simulink model "Exp10"  (R2018a)
settings: Solver=ode23tb  StartTime=0.0  StopTime=0.4  RelTol=1e-4
libraries: powerlib x31
Description:
  | Copyright 2008-2018 The MathWorks, Inc.
settings Model: ExtModeTrigMode=oneshot  ExtModeArmWhenConnect=off  ExtModeAutoUpdateStatusClock=off  Creator=MathWorks  LastModifiedBy=Asus
settings DataIOCC: ExternalInput=[]  SaveFormat=Array  SignalLoggingSaveFormat=ModelDataLogs  SaveOutput=off  SignalLoggingName=sigsOut
settings OptimizationCC: BlockReduction=off  BooleanDataType=off  ExpressionDepthLimit=2147483647  InitFltsAndDblsToZero=on  EfficientMapNaN2IntZero=off  LifeSpan=inf
settings DebuggingCC: AlgebraicLoopMsg=none  UnderspecifiedInitializationDetection=Classic  MergeDetectMultiDrivingBlocksExec=none  CheckExecutionContextPreStartOutputMsg=on  CheckExecutionContextRuntimeOutputMsg=on  SignalResolutionControl=TryResolveAllWithWarning  MultiTaskDSMMsg=warning  MultiTaskCondExecSysMsg=none  SigSpecEnsureSampleTimeMsg=none  FcnCallInpInsideContextMsg=warning  StateNameClashWarn=warning  SFUnexpectedBacktrackingDiag=warning  SFNoUnconditionalDefaultTransitionDiag=warning  SFExecutionAtInitializationDiag=none
settings HardwareCC: ProdBitPerPointer=32  ProdBitPerSizeT=32  ProdBitPerPtrDiffT=32  ProdLargestAtomicFloat=None  ProdIntDivRoundTo=Undefined  ProdEndianess=Unspecified  ProdWordSize=32  ProdHWDeviceType=32-bit Generic  TargetUnknown=on
settings ModelReferenceCC: PropagateSignalLabelsOutOfModel=off
settings CodeAppCC: StateflowObjectComments=on
settings GRTTargetCC: TargetLangStandard=C89/C90 (ANSI)  GeneratePreprocessorConditionals=Disable all  CombineOutputUpdateFcns=off  GRTInterface=on
settings ConfigComp: CovMetricSettings=dw  CovHtmlReporting=on  CovSaveCumulativeToWorkspaceVar=on  CovSaveSingleToWorkspaceVar=on  CovExternalEMLEnable=off  CovSFcnEnable=off
settings SimscapeCC: SimscapeNormalizeSystem=off

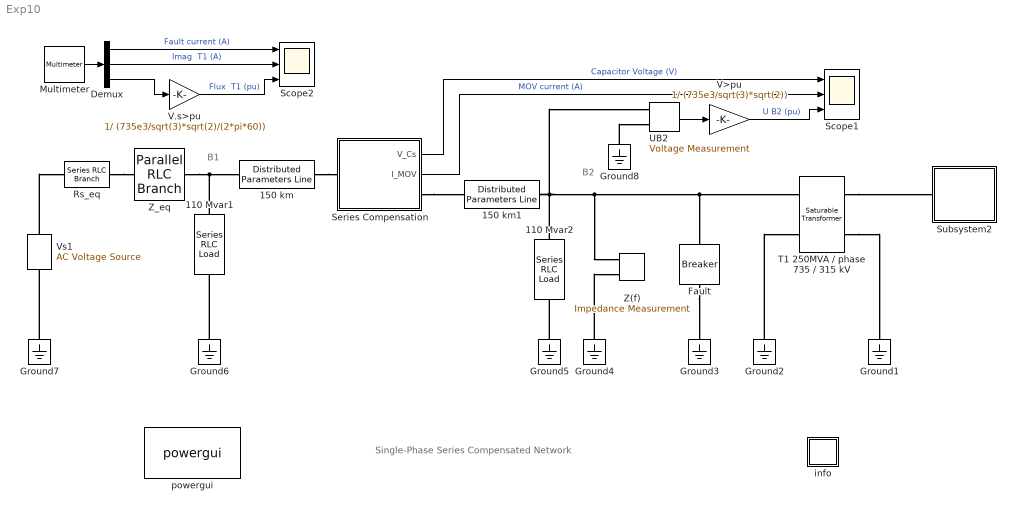
== system Exp10 ==
  note: Single-Phase Series Compensated Network
  note: B1
  note: B2
  110 Mvar1 : powerlib/Elements/Series RLC Load  LConnTagsString=a  RConnTagsString=__new0  NominalVoltage=735000/sqrt(3)  NominalFrequency=60  ActivePower=110e6/300  InductivePower=110e6  CapacitivePower=0  Setx0=off  InitialVoltage=0  SetiL0=off  InitialCurrent=0  Measurements=None  LoadType=constant Z
  110 Mvar2 : powerlib/Elements/Series RLC Load  LConnTagsString=a  RConnTagsString=__new0  NominalVoltage=735000/sqrt(3)  NominalFrequency=60  ActivePower=110e6/300  InductivePower=110e6  CapacitivePower=0  Setx0=off  InitialVoltage=0  SetiL0=off  InitialCurrent=0  Measurements=None  LoadType=constant Z
  150 km : powerlib/Elements/Distributed Parameters Line  Phases=1  Frequency=60  Resistance=0.011  Inductance=0.8674e-03  Capacitance=13.41e-09  Length=150  x1=[602382.210728082;376.991118430775;-0.201832804872111]  x2=[617832.687776944;376.991118430775;-0.223349800057888]  x3=[2166.90364173997;376.991118430775;-0.458497477125126]  x4=[2673.14981372514;376.991118430775;-0.188540324238639]  x5=0.000511582119507709  V1=[6.024e+05;377;-0.2018]  V2=[6.178e+05;377;-0.2233]  I1=[2167;377;-0.4585]  I2=[2673;377;-0.1885]  nHarmo=1  Measurements=None
      settings: AttributesFormatString=\n  SourceProductName=Simscape Power Systems
  150 km1 : powerlib/Elements/Distributed Parameters Line  Phases=1  Frequency=60  Resistance=0.011  Inductance=0.8674e-03  Capacitance=13.41e-09  Length=150  x1=[614251.726505356;376.991118430775;-0.207067226534412]  x2=[606916.918046152;376.991118430775;-0.227269187006359]  x3=[2149.77581818931;376.991118430775;-0.248424449769665]  x4=[2658.79697353536;376.991118430775;-0.366457341038554]  x5=0.000511582119507709  V1=[6.143e+05;377;-0.2071]  V2=[6.069e+05;377;-0.2273]  I1=[2150;377;-0.2484]  I2=[2659;377;-0.3665]  nHarmo=1  Measurements=None
      settings: AttributesFormatString=\n  SourceProductName=Simscape Power Systems
  Demux : Demux  Outputs=3
  Fault : powerlib/Elements/Breaker  InitialState=0  SwitchingTimes="[ 3/60  9/60 ]"  External=off  BreakerResistance=0.01  SnubberResistance=inf  SnubberCapacitance=0  Measurements=Branch current  MoreParameters=off  NoBreakLoop=off
      settings: AttributesFormatString=\n  SourceProductName=Simscape Power Systems
  Ground{1..8} (8 alike) : powerlib/Elements/Ground  LConnTagsString=a
  Multimeter : powerlib/Measurements/Multimeter  Tag=PoWeRsYsTeMmEaSuReMeNt  PhasorSimulation=off  OutputType=Magnitude  sel=[1 3 4]  L=4  Gain=[1 1 1]  yselected="{'Ib: Fault','Imag: T1  250MVA // phase  735 // 315 kV','Flux: T1  250MVA // phase  735 // 315 kV'};"  PSBOutputType=1  PSBequivalent=0  AxesSetting=[0,0.1,-100,100]  Display=0  SavedBlockNames={}
      settings: AttributesFormatString=\n
  Rs_eq : powerlib/Elements/Series RLC Branch  LConnTagsString=__new0  RConnTagsString=__new0  BranchType=R  Resistance=2  Inductance=[]  SetiL0=off  InitialCurrent=0  Capacitance=[]  Setx0=off  InitialVoltage=0  Measurements=None
  Scope1 : Scope  NumInputPorts=3
  Scope2 : Scope  NumInputPorts=3
  Series Compensation : Subsystem
      mask Display: plot(0,0,100,100,[10 40],[50 50], [40 40],[40 60],[60 60],[40 60], [60 90],[50 50])
  Subsystem2 : Subsystem
      mask Display: disp('315 kV\nEquivalent')
  T1 250MVA / phase 735 / 315 kV : powerlib/Elements/Saturable Transformer  ThreeWindings=off  Hysteresis=off  DataFile='hysteresis'  Measurements=Flux and magnetization current ( Imag )  UNITS=pu  NominalPower=[750e6/3,60]  Winding1=[735000/sqrt(3), 0.001 ,0.15]  Winding2=[315000/sqrt(3), 0.001,0]  Winding3=[315000/sqrt(3), 0.001,0]  Saturation=[0 0 ; 0.0012 1.2; 1.0 1.45 ]  CoreLoss=[1000]  MoreParameters=off  BreakLoop=off  DataType=off  InitialFlux=-1606.09832312951  TransfoNumber=1
      settings: AttributesFormatString=\n  SourceProductName=Simscape Power Systems  SourceProductBaseCode=PS
  UB2 : powerlib/Measurements/Voltage Measurement  Tag=PoWeRsYsTeMmEaSuReMeNt  PhasorSimulation=off  OutputType=Magnitude  PSBequivalent=0
  V.s>pu : Gain  Gain=1/ (735e3/sqrt(3)*sqrt(2)/(2*pi*60))  SaturateOnIntegerOverflow=on  OutDataTypeStr=Inherit: Same as input  ParamDataTypeStr=Inherit: Same as input
  V>pu : Gain  Gain=1/ (735e3/sqrt(3)*sqrt(2))  SaturateOnIntegerOverflow=on  OutDataTypeStr=Inherit: Same as input  ParamDataTypeStr=Inherit: Same as input
  Vs1 : powerlib/Electrical Sources/AC Voltage Source  Description=source block  Amplitude=735000/sqrt(3)*sqrt(2)  Phase=0  Frequency=60  SampleTime=0  Measurements=None  BusType=swing  Pref=10e3  Qref=0  Qmin=-inf  Qmax=+inf
      settings: AttributesFormatString=\n
  Z(f) : powerlib/Measurements/Impedance Measurement  LConnTagsString=+|-  Factor=1
      settings: AttributesFormatString=\n  SourceProductName=Simscape Power Systems  SourceProductBaseCode=PS
  Z_eq : powerlib/Elements/Parallel RLC Branch  LConnTagsString=a  RConnTagsString=__new0  BranchType=RLC  Resistance=180.1  Inductance=.026525  SetiL0=off  InitialCurrent=0  Capacitance=117.84e-06  Setx0=off  InitialVoltage=0  Measurements=None
  info : Subsystem
      settings: OpenFcn=showdemo(bdroot(gcb))
      mask Display: disp('?')
  powergui : powerlib/powergui  Priority=2  SimulationMode=Continuous  SampleTime=0  frequency=60  Iterations=50  frequencyindice=60  Pbase=100e6  ErrMax=1e-4  UnitsV=kV  UnitsW=MW  buscounter=0  FunctionMessages=off  echomessages=off  EnableUseOfTLC=off  CurrentSourceSwitches=off  DisableSnubberDevices=on  DisableRonSwitches=off  DisableVfSwitches=off  DisplayEquations=off  SolverType=Tustin  Interpol=off  ExternalGateDelay=off  methode=off  Ts=0  x0status=blocks  SPID=on  SwTol=0  HookPort=off  RestoreLinks=warning  ResistiveCurrentMeasurement=off  Frange=0:500  Ylog=off  Xlog=off  ShowGrid=off  save=off  variable=ZData  structure=0  ZoomFFT=on  StartTime=0.0  cycles=2  DisplayStyle=off  fundamental=60  FreqAxis=off  MaxFrequency=1000  frequencyindicesteady=1  RmsSteady=1  display=off
  wires:
  V>pu/1 -> Scope1/3  "U B2 (pu)"
  Demux/3 -> V.s>pu/1
  Demux/1 -> Scope2/1  "Fault current (A)"
  V.s>pu/1 -> Scope2/3  "Flux  T1 (pu)"
  Demux/2 -> Scope2/2  "Imag  T1 (A)"
  Multimeter/1 -> Demux/1
  UB2/1 -> V>pu/1
  Series Compensation/1(V_Cs) -> Scope1/1  "Capacitor Voltage (V)"
  Series Compensation/2(I_MOV) -> Scope1/2  "MOV current (A)"
  connections:
  T1 250MVA / phase 735 / 315 kV/RConn2 -- Ground1/LConn1
  Ground2/LConn1 -- T1 250MVA / phase 735 / 315 kV/LConn2
  Fault/RConn1 -- Ground3/LConn1
  Ground6/LConn1 -- 110 Mvar1/LConn1
  Ground7/LConn1 -- Vs1/LConn1
  Vs1/RConn1 -- Rs_eq/LConn1
  Z_eq/RConn1 -- 150 km/LConn1 -- 110 Mvar1/RConn1
  Ground5/LConn1 -- 110 Mvar2/LConn1
  T1 250MVA / phase 735 / 315 kV/RConn1 -- Subsystem2/LConn1
  Ground4/LConn1 -- Z(f)/LConn2
  150 km/RConn1 -- Series Compensation/LConn1
  Rs_eq/RConn1 -- Z_eq/LConn1
  150 km1/RConn1 -- 110 Mvar2/RConn1 -- UB2/LConn1 -- T1 250MVA / phase 735 / 315 kV/LConn1 -- Fault/LConn1 -- Z(f)/LConn1
  Ground8/LConn1 -- UB2/LConn2
  Series Compensation/RConn1 -- 150 km1/LConn1

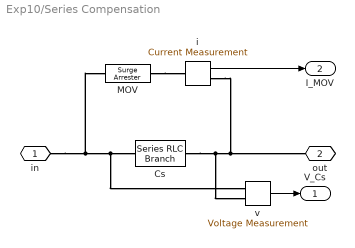
== system Exp10/Series Compensation ==
  Cs : powerlib/Elements/Series RLC Branch  LConnTagsString=__new0  RConnTagsString=__new0  BranchType=C  Resistance=[]  Inductance=[]  SetiL0=off  InitialCurrent=0  Capacitance=67.6e-6  Setx0=off  InitialVoltage=0  Measurements=None
  MOV : powerlib/Elements/Surge Arrester  ProtectionVoltage=277e+03  Columns=30  ReferenceCurrent=500  Segment1=[.955 50]  Segment2=[1.0 25]  Segment3=[.9915 16.5]  Measurements=None  BreakLoop=on
      settings: AttributesFormatString=\n  SourceProductName=Simscape Power Systems  SourceProductBaseCode=PS
  i : powerlib/Measurements/Current Measurement  Tag=PoWeRsYsTeMmEaSuReMeNt  PhasorSimulation=off  OutputType=Magnitude  PSBequivalent=0
  v : powerlib/Measurements/Voltage Measurement  Tag=PoWeRsYsTeMmEaSuReMeNt  PhasorSimulation=off  OutputType=Magnitude  PSBequivalent=0
  in : PMIOPort  Side=Left
  out : PMIOPort  Port=2  Side=Right
  V_Cs : Outport
  I_MOV : Outport  Port=2
  wires:
  i/1 -> I_MOV/1
  v/1 -> V_Cs/1
  connections:
  in/RConn1 -- Cs/LConn1 -- v/LConn1 -- MOV/LConn1
  MOV/RConn1 -- i/LConn1
  Cs/RConn1 -- out/RConn1 -- i/RConn1 -- v/LConn2

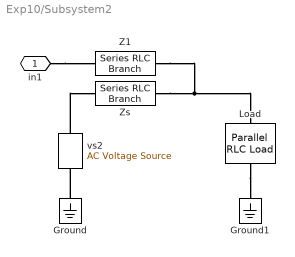
== system Exp10/Subsystem2 ==
  Ground : powerlib/Elements/Ground  LConnTagsString=a
  Ground1 : powerlib/Elements/Ground  LConnTagsString=a
  Load : powerlib/Elements/Parallel RLC Load  LConnTagsString=a  RConnTagsString=__new0  NominalVoltage=315000/sqrt(3)  NominalFrequency=60  ActivePower=200e6  InductivePower=0  CapacitivePower=50e6  Setx0=off  InitialVoltage=0  SetiL0=off  InitialCurrent=0  Measurements=None  LoadType=constant Z
      settings: AttributesFormatString=\n  SourceProductName=Simscape Power Systems  SourceProductBaseCode=PS
  Z1 : powerlib/Elements/Series RLC Branch  LConnTagsString=__new0  RConnTagsString=__new0  BranchType=RL  Resistance=0.734  Inductance=0.02085  SetiL0=off  InitialCurrent=0  Capacitance=[]  Setx0=off  InitialVoltage=0  Measurements=None
  Zs : powerlib/Elements/Series RLC Branch  LConnTagsString=__new0  RConnTagsString=__new0  BranchType=RL  Resistance=11.0  Inductance=0.2925  SetiL0=off  InitialCurrent=0  Capacitance=[]  Setx0=off  InitialVoltage=0  Measurements=None
  vs2 : powerlib/Electrical Sources/AC Voltage Source  Description=source block  Amplitude=315000/sqrt(3)*sqrt(2)  Phase=20  Frequency=60  SampleTime=0  Measurements=None  BusType=swing  Pref=10e3  Qref=0  Qmin=-inf  Qmax=+inf
      settings: AttributesFormatString=\n
  in1 : PMIOPort  Side=Left
  connections:
  Load/RConn1 -- Ground1/LConn1
  Z1/RConn1 -- Load/LConn1 -- Zs/RConn1
  in1/RConn1 -- Z1/LConn1
  vs2/RConn1 -- Zs/LConn1
  Ground/LConn1 -- vs2/LConn1

== system Exp10/info ==
